simulink model "ShoppingCartManagementInterface"  (R2024a)
settings: Solver=FixedStepAuto  StartTime=0.0  StopTime=10.0  RelTol=1e-3
libraries: simulink x1
settings Model: Creator=chico  LastModifiedBy=chico

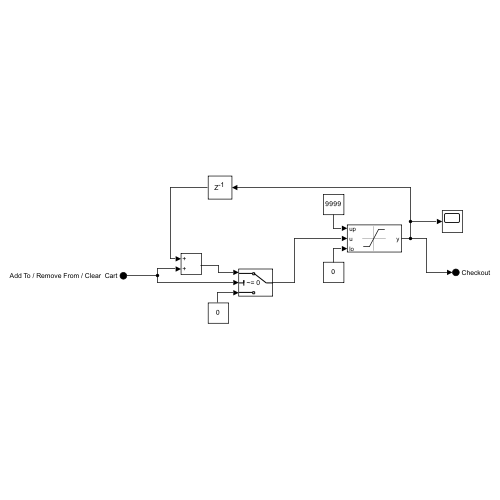
[thumbnail: Simulink's stored preview of the top-level diagram]
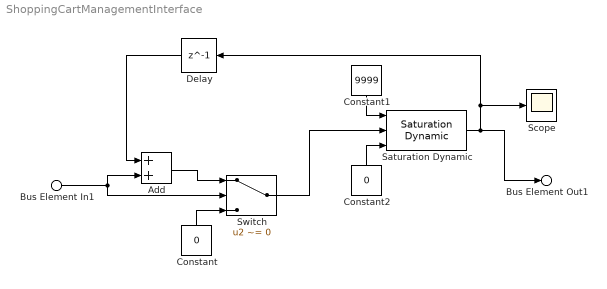
== system ShoppingCartManagementInterface ==
  Bus Element In1 : Inport  PortName="Add To / Remove From / Clear  Cart"
  Add : Sum
  Constant : Constant  Value=0
  Constant1 : Constant  Value=9999
  Constant2 : Constant  Value=0
  Delay : Delay  DelayLength=1
  Saturation Dynamic : simulink/Discontinuities/Saturation Dynamic  OutMin=[]  OutMax=[]  OutDataTypeStr=Inherit: Same as second input  OutDataType=fixdt(1, 16)  OutScaling=2^-10  DoSatur=off
  Scope : Scope
  Switch : Switch  Criteria=u2 ~= 0  SaturateOnIntegerOverflow=off  InputSameDT=off
  Bus Element Out1 : Outport  PortName=Checkout
  wires:
  Bus Element In1/1 -> Switch/2, Add/2
  Delay/1 -> Add/1
  Add/1 -> Switch/1
  Constant/1 -> Switch/3
  Constant1/1 -> Saturation Dynamic/1
  Switch/1 -> Saturation Dynamic/2
  Constant2/1 -> Saturation Dynamic/3
  Saturation Dynamic/1 -> Scope/1, Delay/1, Bus Element Out1/1
